simulink model "PIDDIDIER"  (R2017b)
settings: Solver=VariableStepAuto  StartTime=0.0  StopTime=10.0  RelTol=1e-3
values from neighbouring files (symbols this model uses):
  kd = eval(S.kd)    [Parcial1.m]
  kd2 = eval(S.kd2)    [Parcial1.m]
  ki = eval(Sol.ki)    [PUNTO1PARCIAL.m]    (also in PUNTO1PARCIALLLINTENTO2.m; Parcial1.m = eval(S.ki); parcialretro.m)
  ki2 = eval(Sol.ki2)    [PUNTO1PARCIAL.m]    (also in Parcial1.m = eval(S.ki2); parcialretro.m)
  kp = eval(S.kp)    [Parcial1.m]
libraries: simulink x1
settings Model: Creator=Cx001la  LastModifiedBy=Cx001la

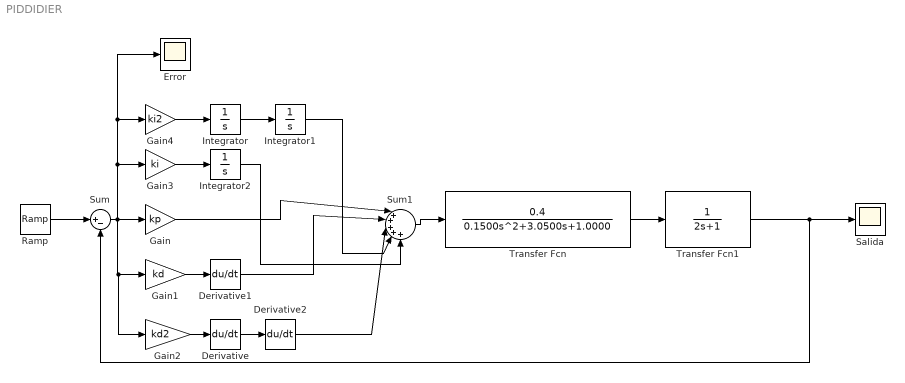
== system PIDDIDIER ==
  Derivative : Derivative
  Derivative1 : Derivative
  Derivative2 : Derivative
  Error : Scope
  Gain : Gain  Gain=kp
  Gain1 : Gain  Gain=kd
  Gain2 : Gain  Gain=kd2
  Gain3 : Gain  Gain=ki
  Gain4 : Gain  Gain=ki2
  Integrator : Integrator
  Integrator1 : Integrator
  Integrator2 : Integrator
  Ramp : simulink/Sources/Ramp  slope=1  start=0  X0=0
  Salida : Scope
  Sum : Sum  Inputs=|+-
  Sum1 : Sum  Inputs=|+++++
  Transfer Fcn : TransferFcn  Numerator=[0.4]  Denominator="[0.1500    3.0500    1.0000]"
  Transfer Fcn1 : TransferFcn  Denominator=[2 1]
  wires:
  Ramp/1 -> Sum/1
  Gain2/1 -> Derivative/1
  Derivative/1 -> Derivative2/1
  Gain1/1 -> Derivative1/1
  Sum/1 -> Gain2/1, Gain1/1, Gain3/1, Gain4/1, Error/1, Gain/1
  Derivative2/1 -> Sum1/3
  Derivative1/1 -> Sum1/2
  Gain/1 -> Sum1/1
  Sum1/1 -> Transfer Fcn/1
  Transfer Fcn/1 -> Transfer Fcn1/1
  Transfer Fcn1/1 -> Salida/1, Sum/2
  Gain3/1 -> Integrator2/1
  Gain4/1 -> Integrator/1
  Integrator/1 -> Integrator1/1
  Integrator2/1 -> Sum1/5
  Integrator1/1 -> Sum1/4
